simulink library "INT_T15_DD"  (R2016b)
settings: Solver=VariableStepAuto  StartTime=0.0  StopTime=10.0  RelTol=1e-3
settings Model: Creator=Administrator  LastModifiedBy=Administrator

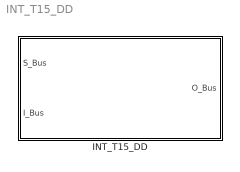
== system INT_T15_DD ==
  INT_T15_DD : Subsystem

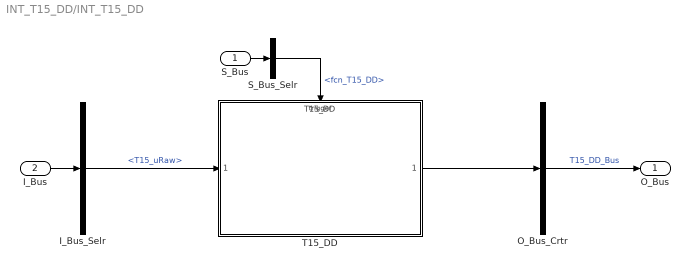
== system INT_T15_DD/INT_T15_DD ==
  S_Bus : Inport
  I_Bus : Inport  Port=2
  I_Bus_Selr : BusSelector  OutputSignals=T15_uRaw
  O_Bus_Crtr : BusCreator  Inputs=1
  S_Bus_Selr : BusSelector  OutputSignals=fcn_T15_DD
  T15_DD : ModelReference  ModelNameDialog=T15_DD  SimulationMode=Normal  ModelReferenceVersion=1.8  TriggerPortName=function  TriggerPortTriggerType=function-call  TriggerPortStatesWhenEnabling=held
  O_Bus : Outport
  wires:
  S_Bus_Selr/1 -> T15_DD/Trigger  "<fcn_T15_DD>"
  S_Bus/1 -> S_Bus_Selr/1
  I_Bus/1 -> I_Bus_Selr/1
  I_Bus_Selr/1 -> T15_DD/1  "<T15_uRaw>"
  O_Bus_Crtr/1 -> O_Bus/1  "T15_DD_Bus"
  T15_DD/1 -> O_Bus_Crtr/1
